simulink model "extractTF"  (R2024a)
settings: Solver=FixedStepDiscrete  StartTime=0.0  StopTime=10.0  RelTol=1e-3  EnableMultiTasking=on
undefined symbols (not defined in the file or in its folder): tag36h11
libraries: ros2lib x2
settings Model: Creator=WHZ-46833  LastModifiedBy=WHZ-46833
settings SolverCC: AutoInsertRateTranBlk=on
settings DataIOCC: SaveOutput=off  SaveTime=off
settings OptimizationCC: DefaultParameterBehavior=Inlined  InlineInvariantSignals=on  EnhancedBackFolding=on  PassReuseOutputArgsAs=Individual arguments  StateBitsets=on  DataBitsets=on  ZeroExternalMemoryAtStartup=off  ZeroInternalMemoryAtStartup=off  NoFixptDivByZeroProtection=on  LifeSpan=1  OptimizeBlockOrder=speed  DifferentSizesBufferReuse=on  EfficientTunableParamExpr=on
settings DebuggingCC: ParameterTunabilityLossMsg=error
settings HardwareCC: ProdBitPerPointer=32  ProdBitPerSizeT=32  ProdBitPerPtrDiffT=32  ProdLargestAtomicFloat=None  ProdIntDivRoundTo=Floor  ProdWordSize=32  ProdHWDeviceType=Generic->Custom
settings SFSimCC: MATLABDynamicMemAlloc=off
settings RTWCC: Description=Embedded Coder  SystemTargetFile=ert.tlc  TLCOptions=-p0  GenCodeOnly=on  TemplateMakefile=ert_default_tmf  GenerateReport=on  RTWVerbose=off  IncludeHyperlinkInReport=on  LaunchReport=on
settings CodeAppCC: ForceParamTrailComments=on  IgnoreCustomStorageClasses=off  OperatorAnnotations=on  SimulinkDataObjDesc=on  SFDataObjDesc=on  CustomSymbolStrGlobalVar=rt$N$M  CustomSymbolStrType=$N$M  CustomSymbolStrFcn=$N$M$F  CustomSymbolStrMacro=$N$M  InsertBlockDesc=on
settings ERTTargetCC: TargetLangStandard=C99 (ISO)  CodeReplacementLibrary=ISO_C  GenerateSampleERTMain=on  IncludeMdlTerminateFcn=off  SuppressErrorStatus=on  SupportAbsoluteTime=off  PurelyIntegerCode=on  SupportNonFinite=off  SupportComplex=off  InlinedParameterPlacement=NonHierarchical  RootIOFormat=Structure reference  ERTCustomFileTemplate=example_file_process.tlc

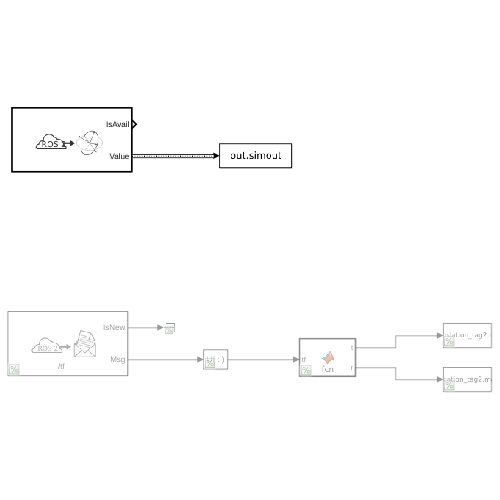
[thumbnail: Simulink's stored preview of the top-level diagram]
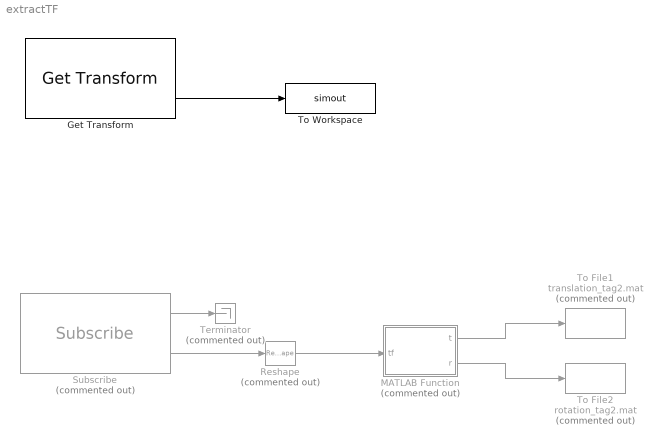
== system extractTF ==
  Get Transform : ros2lib/Get Transform  FrameSource=Select from ROS network  TargetFrame=camera_1  SourceFrame=tag36h11:6  OutputFormat=bus  SampleTime=-1  DynamicQoSHistory=Keep last  DynamicQoSDepth=1  DynamicQoSReliability=Reliable  DynamicQoSDurability=Volatile  DynamicQoSDeadline=Inf  DynamicQoSLifespan=Inf  DynamicQoSLiveliness=Automatic  DynamicQoSLeaseDuration=Inf  DynamicQoSAvoidROSNamespaceConventions=off  StaticQoSHistory=Keep last  StaticQoSDepth=1  StaticQoSReliability=Reliable  StaticQoSDurability=Volatile  StaticQoSDeadline=Inf  StaticQoSLifespan=Inf  StaticQoSLiveliness=Automatic  StaticQoSLeaseDuration=Inf  StaticQoSAvoidROSNamespaceConventions=off
  MATLAB Function : MATLAB Function  Commented=on  TreatAsAtomicUnit=on
  Reshape : Reshape  Commented=on  OutputDimensions=1
  Subscribe : ros2lib/Subscribe  Commented=on  topicSource=Select from ROS network  topic=/tf  messageType=tf2_msgs/TFMessage  sampleTime=-1  QOSHistory=Keep last  QOSDepth=1  QOSReliability=Reliable  QOSDurability=Volatile  QOSDeadline=Inf  QOSLifespan=Inf  QOSLiveliness=Automatic  QOSLeaseDuration=Inf  QOSAvoidROSNamespaceConventions=off
  Terminator : Terminator  Commented=on
  To File1 : ToFile  Commented=on  Filename=translation_tag2.mat  MatrixName=trans  SaveFormat=Timeseries
  To File2 : ToFile  Commented=on  Filename=rotation_tag2.mat  MatrixName=rot  SaveFormat=Timeseries
  To Workspace : ToWorkspace  VariableName=simout  SaveFormat=Timeseries  SampleTime=-1
  wires:
  MATLAB Function/1(t) -> To File1/1
  MATLAB Function/2(r) -> To File2/1
  Subscribe/1 -> Terminator/1
  Subscribe/2 -> Reshape/1
  Reshape/1 -> MATLAB Function/1(tf)
  Get Transform/2 -> To Workspace/1

== matlab function extractTF/MATLAB Function ==
  data: tf input; t output; r output
function [t, r]= fcn(tf)
%tftree = tf;
tagtocamera = getTransform(tf, 'tag36h11:2', 'camera_1');
t = tagtocamera.Transform.Translation;
r = tagtocamera.Transform.Rotation;
end
